simulink model "d_lab"  (R2024a)
settings: Solver=VariableStepAuto  StartTime=0.0  StopTime=10  RelTol=1e-6
undefined symbols (not defined in the file): A, B, C, D
settings Model: Creator=lenovo  LastModifiedBy=lenovo

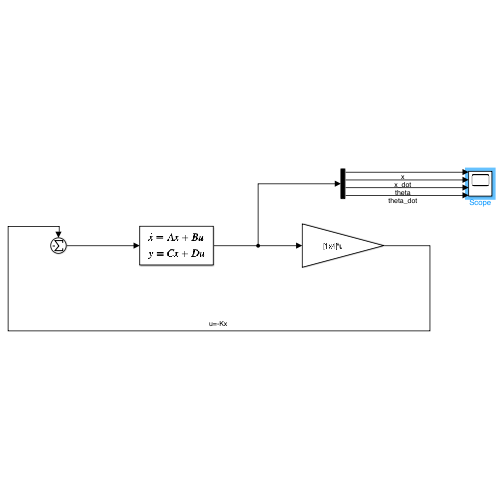
[thumbnail: Simulink's stored preview of the top-level diagram]
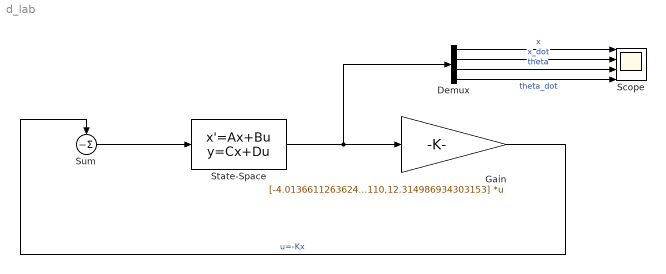
== system d_lab ==
  Demux : Demux
  Gain : Gain  Gain=[-4.013661126362421,-6.096942377664535,50.954581395955110,12.314986934303153]  Multiplication=Matrix(K*u)
  Scope : Scope  NumInputPorts=4
  State-Space : StateSpace  A=A  B=B  C=C  D=D  InitialCondition=[0.2; 0; 0.2; 0]
  Sum : Sum  Inputs=-|
  wires:
  State-Space/1 -> Demux/1, Gain/1
  Demux/1 -> Scope/1  "x"
  Demux/2 -> Scope/2  "x_dot"
  Demux/3 -> Scope/3  "theta"
  Demux/4 -> Scope/4  "theta_dot"
  Sum/1 -> State-Space/1
  Gain/1 -> Sum/1  "u=-Kx"
